simulink model "Inverter_SPI"  (R2018b)
settings: Solver=FixedStepAuto  StartTime=tsim_start  StopTime=tsim_end  FixedStep=1  RelTol=1e-3
undefined symbols (not defined in the file): ActPower1, ActPower2, ActPower3, path_carnot, phase, soc0, socMax, socMin, Tstest
settings Model: SimulationMode=accelerator  PauseTimes=36459  Creator=P41573  LastModifiedBy=P41573
settings DataIOCC: ReturnWorkspaceOutputs=on
settings OptimizationCC: EfficientMapNaN2IntZero=off
settings HardwareCC: TargetBitPerPointer=64  TargetBitPerSizeT=64  TargetBitPerPtrDiffT=64  TargetLongLongMode=on  TargetIntDivRoundTo=Zero  TargetEndianess=LittleEndian  TargetWordSize=64  TargetHWDeviceType=MATLAB Host  ProdEqTarget=off
settings CodeAppCC: MaxIdLength=128
settings GRTTargetCC: TargetLangStandard=C89/C90 (ANSI)  CombineOutputUpdateFcns=off  GRTInterface=on

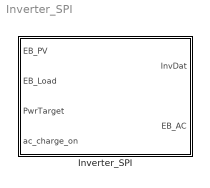
== system Inverter_SPI ==
  Inverter_SPI : Subsystem  mask(Inverter_SPI){PathName=fullfile(path_carnot('libsl'), 'Source', 'Electric_Generator', 'Inverter_SPI', 'parameter_set'), FileName='Kostal_Plenticicore_5p5_BatterBox_H11p5.mat', userPath=off, userParam=off, nphase=3-phase, soc0=soc0, socMin=socMin, socMax=socMax, Tsample=Tstest, capUser=0, SpiData=[5.686;5.487;6.35626283367556;6.191;5.419;0;73.4437227313543;94.5955883042527;31.1212070123701;74.9053455860837;92.4754002317794;31.7469866284786;30.8769273130404;90.5542640263268;41.6993897221684;86.4449570278825;105.13781756438;31.4770198650726;1;1;1;1;1;1;0.98;0.98;1.32333333333333;0.15;0;4.47;4.56;1.55;10.7670579897002;95.2833]}
      mask prompts: PathName "Path"; FileName "Parameter set"; userPath "Edit path and name of parameter set"; userParam "User defined parameters"; nphase "Number of phases"; soc0 "Initial State of Charge (0..1)"; socMin "Min. State of Charge (0..1)"; socMax "Max. State of Charge (0..1)"; Tsample "Sample Time (default =1s) [s]"; capUser "Battery capacity  (<=0 for default) [kWh]"; SpiData "SPI Parameter Set"
      mask help:
      | Hybrid Inverter with DC Battery
      | Efficiency of all power pahts is calculated by quadratic loss equation. Simple control dynamics are implemented as PT1 behavior.
      | This model is a simulink conversion of PermodDC Model by HTW Berlin.
      mask init:
      | % callback to set parameters of model
      | [ok, param] = CarnotCallbacks_Inverter_SPI('SetParameters',gcbh,PathName,FileName);
      mask Help: web(fullfile(path_carnot('help'),'Inverter_SPI.html'),'-helpbrowser')
      mask Callback userPath: [ok, param] = CarnotCallbacks_Inverter_SPI('UserEdit',gcbh);
      mask Callback userParam: [ok, param] = CarnotCallbacks_Inverter_SPI('UserEdit',gcbh);
      mask TypeOptions nphase: Nphase/nphase
      mask TypeOptions soc0: S-Function/soc0
      mask TypeOptions socMin: S-Function/soc_min
      mask TypeOptions socMax: S-Function/soc_max
      mask TypeOptions Tsample: S-Function/inv_Ts
      mask TypeOptions capUser: S-Function/cap_user
      mask TypeOptions SpiData: S-Function/spi_data
      mask DialogControl ParameterGroupFile Prompt: Picking a parameter set
      mask DialogControl Control2 Prompt: Carnot public data
      mask DialogControl Control2 Callback: [ok, file] = CarnotCallbacks_Inverter_SPI('GetFilename',gcbh,'public');
      mask DialogControl Control3 Prompt: Carnot internal data
      mask DialogControl Control3 Callback: [ok, file] = CarnotCallbacks_Inverter_SPI('GetFilename',gcbh,'internal');
      mask DialogControl Control4 Prompt: Selected path
      mask DialogControl Control4 Callback: [ok, file] = CarnotCallbacks_Inverter_SPI('GetFilename',gcbh,'selected');
      mask DialogControl Container7 Prompt: Parameters
      mask Display:
      | pic = false;
      | if ~BlockIsInCarnotLibrary    % if not located in library any more
      |     picfile = fullfile(path_carnot('intlibsl'), ...
      |         'Source','Electric_Generator','Inverter_SPI','parameter_set', ...
      |         'Inverter_SPI.jpg');
      |     if exist(picfile,'file') % show internal picture if defined
      |         image(imread(picfile), [0.2, 0, 0.6, 1])
      |         set_param(gcb, 'BackgroundColor', 'White')
      |         pic = true;
      |     end
      | end
      | if ~pic    % show public picture
      |     set_param(gcb, 'BackgroundColor', 'Orange')
      |     xo=0;
      |     plot(0,0,100,100,...
      |         xo+[76,30,76,76,30,30],[45,95,95,45,45,95],...
      |         xo+[35,45],[60,60],[35,45],[55,55],...
      |         xo+[73,71,67,63,59,57],[80,75,75,85,85,80],...
      |         xo+[76,30,30,76,76],[5,5,35,35,5],...)
      |         [53,53],[35,45],[55,55],[35,45],...
      |         [38.5,41.5],[30,30],[40,40],[28,32],xo+[64,68],[30,30])
      | end

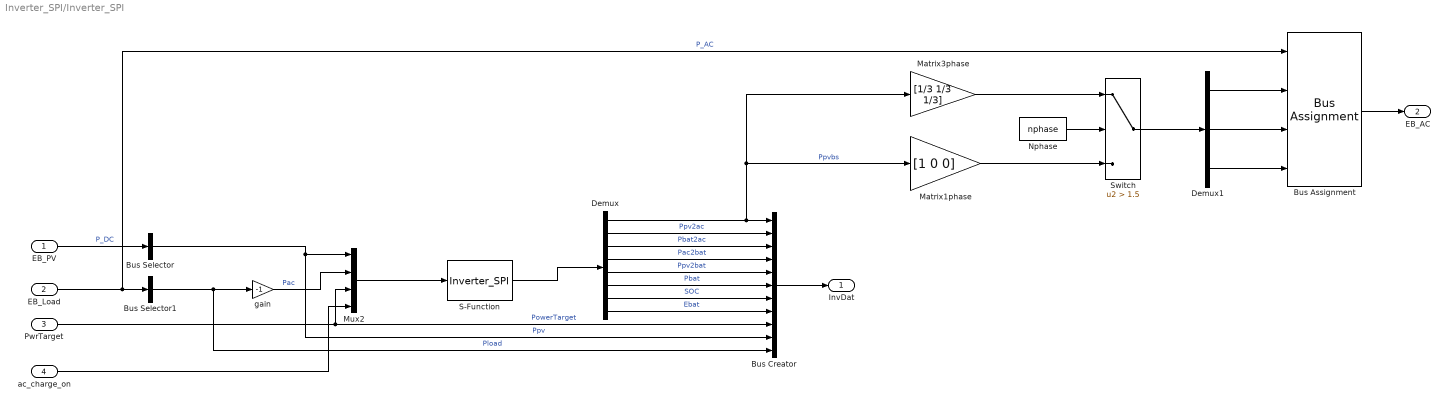
== system Inverter_SPI/Inverter_SPI ==
  EB_PV : Inport
  EB_Load : Inport  Port=2
  PwrTarget : Inport  Port=3  Unit=W
  ac_charge_on : Inport  Port=4  Unit=W
  Bus Assignment : BusAssignment  AssignedSignals=ActPower1,ActPower2,ActPower3
  Bus Creator : BusCreator  Inputs=11
  Bus Selector : BusSelector  OutputSignals=ActPower1  OutputAsBus=on
  Bus Selector1 : BusSelector  OutputSignals=ActPower1  OutputAsBus=on
  Demux : Demux  Outputs=8
  Demux1 : Demux  Outputs=3
  Matrix1phase : Gain  Gain=[1 0 0]
  Matrix3phase : Gain  Gain=[1/3 1/3 1/3]
  Mux2 : Mux
  Nphase : Constant  Value=nphase  mask{nphase=3-phase}
      mask prompts: nphase "Number of phases"
      mask TypeOptions nphase: 1-phase | 3-phase
  S-Function : S-Function  FunctionName=Inverter_SPI  Parameters=soc0,cap_user,soc_min,soc_max,spi_data, inv_Ts  SFunctionDeploymentMode=off  EnableBusSupport=off  mask{spi_data=SpiData, soc0=soc0, soc_min=socMin, soc_max=socMax, inv_Ts=Tsample, cap_user=capUser}
      mask prompts: spi_data "SPI Parameters"; soc0 "initial state of charge"; soc_min "minimum  state of charge"; soc_max "maximum state of charge"; inv_Ts "sample Time"; cap_user "override battery capacity"
      mask init:
      | if isempty(spi_data)
      |    spi_data = [5;5;4;4;4;5;0;0;0;0;0;0;0;0;0;0;0;0;0;0;0;0;0;0;0.980000000000000;2;5;0;0;0;0;1;5;90] 
      | end
      | if isempty(soc0)
      |    soc0 = 0;
      | end
      | if isempty(soc_min)
      |    soc_min = 0;
      | end
      | if isempty(soc_max)
      |    soc_max = 0;
      | end
      | if isempty(inv_Ts)
      |    inv_Ts = 1;
      | end
      | if isempty(cap_user)
      |    cap_user = 0;
      | end
  Switch : Switch  Criteria=u2 > Threshold  Threshold=1.5
  gain : Gain  Gain=-1
  InvDat : Outport
  EB_AC : Outport  Port=2
  wires:
  ac_charge_on/1 -> Mux2/4
  Bus Selector1/1 -> Bus Creator/11, gain/1  "Pload"
  Switch/1 -> Demux1/1
  Matrix1phase/1 -> Switch/3
  Matrix3phase/1 -> Switch/1
  Nphase/1 -> Switch/2
  Demux1/3 -> Bus Assignment/4
  Bus Assignment/1 -> EB_AC/1
  Demux1/2 -> Bus Assignment/3
  Demux1/1 -> Bus Assignment/2
  EB_Load/1 -> Bus Assignment/1, Bus Selector1/1  "P_AC"
  S-Function/1 -> Demux/1
  Demux/1 -> Matrix1phase/1, Matrix3phase/1, Bus Creator/1  "Ppvbs"
  Bus Selector/1 -> Mux2/1, Bus Creator/10  "Ppv"
  Bus Creator/1 -> InvDat/1
  Demux/5 -> Bus Creator/5  "Ppv2bat"
  gain/1 -> Mux2/2  "Pac"
  Demux/7 -> Bus Creator/7  "SOC"
  Demux/4 -> Bus Creator/4  "Pac2bat"
  Demux/6 -> Bus Creator/6  "Pbat"
  PwrTarget/1 -> Bus Creator/9, Mux2/3  "PowerTarget"
  Demux/3 -> Bus Creator/3  "Pbat2ac"
  Mux2/1 -> S-Function/1
  Demux/2 -> Bus Creator/2  "Ppv2ac"
  Demux/8 -> Bus Creator/8  "Ebat"
  EB_PV/1 -> Bus Selector/1  "P_DC"
